simulink model "Auris_ES14"  (R2019a)
settings: Solver=FixedStepAuto  StartTime=0.0  StopTime=10000  FixedStep=.1  RelTol=1e-5
PostLoadFcn:
  | if builtin('license','test','virtual_reality_toolbox')
  |     set_param([gcs '/Simulink 3D Animation'], 'enableVis', 'on')
  | else
  |     set_param([gcs '/Simulink 3D Animation'], 'enableVis', 'off')
  | end
InitFcn:
  | if strcmp(get_param([gcs '/Simulink 3D Animation'], 'enableVis'), 'on')
  |     if ~builtin('license','checkout','virtual_reality_toolbox')
  |         error(message('aeroblks_cubesat:cubesat:licenseFailAnimTemplate'));
  |     end
  | end
model workspace (MATLAB code in the model file + MAT data in the model file):
  aeroCoeff : struct (value not decoded)
  environment : struct (value not decoded)
  initCond : struct (value not decoded)
  inputs0 : struct (value not decoded)
  states0 : struct (value not decoded)
  vehicle : struct (value not decoded)
  other statements: initialize6DOFSkyHogg;
values from neighbouring files (symbols this model uses):
  combine_x_std = sqrt(sum([combine_x_std, pos_unc].^2))    [Pointing_Budget.m]
  combine_y_std = sqrt(sum([combine_y_std, pos_unc].^2))    [Pointing_Budget.m]
  combine_z_std = sqrt(sum([combine_z_std, pos_unc].^2))    [Pointing_Budget.m]
  epoch = juliandate(tle.epoch.year, 1, 1) + tle.epoch.day * 86400    [ADC_Sim_init.m]
  inertia = inertia * conversion    [ADC_Sim_init.m]
  initial_ang_rate = [0, 0, 0]    [ADC_Sim_init.m]
  initial_euler = [0, 0, 180]    [ADC_Sim_init.m]
  s = line1(3:7)    [read_tloes.m]
  semi_major = (((86400 / tle.mean_motion) / (2 * pi))^2 * 398.6e12)^(1 / 3)    [ADC_Sim_init.m]
  starting_time = juliandate(date)    [ADC_Sim_init.m]
  tle = read_tloes('ISS_TLE.txt')    [ADC_Sim_init.m]
  true_anomaly = tle.mean_anomaly + (2 * exp(1) - 1 / 4 * exp(3)) * sind(tle.mean_anomaly) + 5 / 4 * exp(2) * sind(2 * tle.mean_anomaly) + 13/12 * exp(3) * sind(3 * tle.mean_anomaly)    [ADC_Sim_init.m]
undefined symbols (not defined in the file or in its folder): constraintAxes, Earth, euler0, IAU, km, pointing, pqr0, WGS84
libraries: aerolibutil x19, vrlib x8, aerolibconvert2 x6, sharedtransform x5, aerolibtransform2 x5, aerolibcelestial x3, asbCubeSatBlockLib x2, simulink x2, simulink_extras x2, aerolib6dof2 x1, sharedutil x1, aerolibobsolete x1
(part 2 of 2)

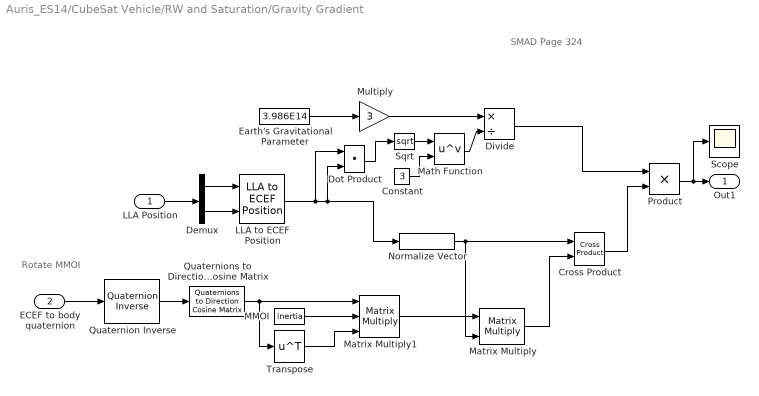
== system Auris_ES14/CubeSat Vehicle/RW and Saturation/Gravity Gradient ==
  note: SMAD Page 324
  note: Rotate MMOI
  LLA Position : Inport
  ECEF to body quaternion : Inport  Port=2
  Constant : Constant  Value=3
  Cross Product : vrlib/Utilities/Cross Product
      settings: SourceProductName=Simulink
  Demux : Demux  Outputs=2
  Divide : Product  Inputs=*/
  Dot Product : DotProduct  InputSameDT=on  OutDataTypeStr=Inherit: Inherit via internal rule
  Earth's Gravitational Parameter : Constant  Value=3.986E14
  LLA to ECEF Position : aerolibtransform2/LLA to ECEF Position  units=Metric (MKS)  ptype=Earth (WGS84)  F=1/298.257223563  R=6378137
      settings: SourceProductName=Aerospace Blockset  SourceProductBaseCode=AE
  MMOI : Constant  Value=inertia
  Math Function : Math  Operator=pow  SaturateOnIntegerOverflow=on
  Matrix Multiply : Product  Multiplication=Matrix(*)
  Matrix Multiply1 : Product  Inputs=3  Multiplication=Matrix(*)
  Multiply : Gain  Gain=3
  Normalize Vector : vrlib/Utilities/Normalize Vector  maxzero=0
      settings: SourceProductName=Simulink
  Product : Product
  Quaternion Inverse : aerolibutil/Quaternion Inverse
      settings: SourceProductName=Aerospace Blockset
  Quaternions to Direction Cosine Matrix : sharedtransform/Quaternions to  Direction Cosine Matrix  aMode=aMode
      settings: SourceProductName=Aerospace Blockset  SourceProductBaseCode=AE
  Scope : Scope
  Sqrt : Sqrt  SaturateOnIntegerOverflow=on
  Transpose : Math  Operator=transpose  SaturateOnIntegerOverflow=on
  Out1 : Outport
  wires:
  Demux/1 -> LLA to ECEF Position/1
  Demux/2 -> LLA to ECEF Position/2
  LLA Position/1 -> Demux/1
  Earth's Gravitational Parameter/1 -> Multiply/1
  LLA to ECEF Position/1 -> Normalize Vector/1, Dot Product/2, Dot Product/1
  Math Function/1 -> Divide/2
  Multiply/1 -> Divide/1
  Normalize Vector/1 -> Matrix Multiply/2, Cross Product/1
  Product/1 -> Scope/1, Out1/1
  Divide/1 -> Product/1
  Cross Product/1 -> Product/2
  Matrix Multiply/1 -> Cross Product/2
  ECEF to body quaternion/1 -> Quaternion Inverse/1
  Quaternion Inverse/1 -> Quaternions to Direction Cosine Matrix/1
  MMOI/1 -> Matrix Multiply1/2
  Quaternions to Direction Cosine Matrix/1 -> Transpose/1, Matrix Multiply1/1
  Transpose/1 -> Matrix Multiply1/3
  Matrix Multiply1/1 -> Matrix Multiply/1
  Dot Product/1 -> Sqrt/1
  Sqrt/1 -> Math Function/1
  Constant/1 -> Math Function/2

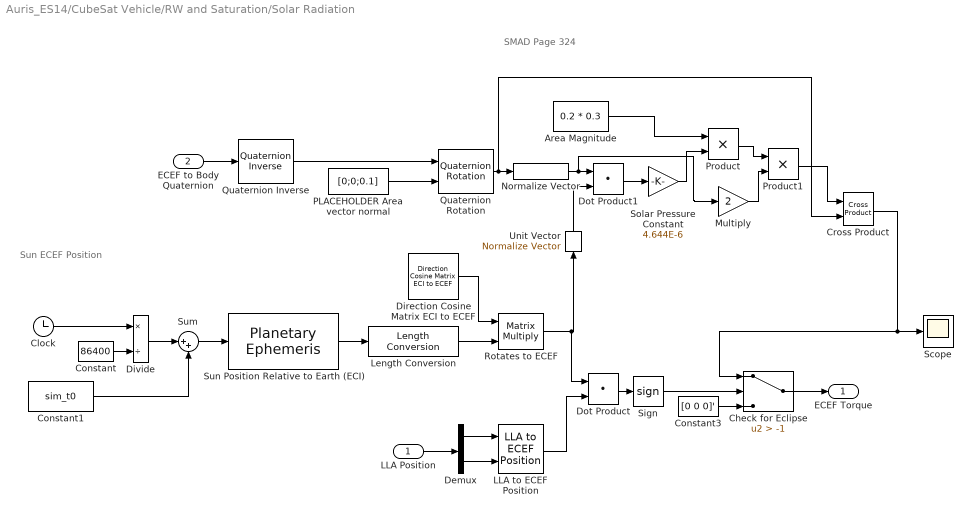
== system Auris_ES14/CubeSat Vehicle/RW and Saturation/Solar Radiation ==
  note: Sun ECEF Position
  note: SMAD Page 324
  LLA Position : Inport
  ECEF to Body Quaternion : Inport  Port=2
  "Area Magnitude " : Constant  Value=0.2 * 0.3
  Check for Eclipse : Switch  Criteria=u2 > Threshold  Threshold=-1
  Clock : Clock
  Constant : Constant  Value=86400
  Constant1 : Constant  Value=sim_t0
  Constant3 : Constant  Value=[0 0 0]'  OutDataTypeStr=Inherit: Inherit via back propagation
  Cross Product : vrlib/Utilities/Cross Product
      settings: SourceProductName=Simulink
  Demux : Demux  Outputs=2
  Direction Cosine Matrix ECI to ECEF : aerolibtransform2/Direction Cosine Matrix ECI to ECEF  red=IAU-2000/2006  year=2019  month=January  day=4  hour=0  min=0  sec=0  deltaT=None  errorflag=Error  extraparamflag=off
      settings: AttributesFormatString=%<red>  SourceProductName=Aerospace Blockset  SourceProductBaseCode=AE
  Divide : Product  Inputs=*/
  Dot Product : DotProduct  InputSameDT=on  OutDataTypeStr=Inherit: Inherit via internal rule
  Dot Product1 : DotProduct  InputSameDT=on  OutDataTypeStr=Inherit: Inherit via internal rule
  LLA to ECEF Position : aerolibtransform2/LLA to ECEF Position  units=Metric (MKS)  ptype=Earth (WGS84)  F=1/298.257223563  R=6378137
      settings: SourceProductName=Aerospace Blockset  SourceProductBaseCode=AE
  Length Conversion : aerolibconvert2/Length Conversion  IU=km  OU=m
  Multiply : Gain  Gain=2
  Normalize Vector : vrlib/Utilities/Normalize Vector  maxzero=0
      settings: SourceProductName=Simulink
  PLACEHOLDER Area vector normal : Constant  Value=[0;0;0.1]
  Product : Product
  Product1 : Product
  Quaternion Inverse : aerolibutil/Quaternion Inverse
      settings: SourceProductName=Aerospace Blockset
  Quaternion Rotation : aerolibutil/Quaternion Rotation
  Rotates to ECEF : Product  Multiplication=Matrix(*)
  Scope : Scope
  Sign : Signum
  Solar Pressure Constant : Gain  Gain=4.644E-6
  Sum : Sum  Inputs=|++
  Sun Position Relative to Earth (ECI) : aerolibcelestial/Planetary Ephemeris  kmflag=km,km/s  epochflag=Julian date  de=DE421  nCenter=Earth  nTarget=Sun  errorflag=Error  velflag=off
      settings: SourceProductName=Aerospace Blockset  SourceProductBaseCode=AE
  Unit Vector : vrlib/Utilities/Normalize Vector  maxzero=0
      settings: SourceProductName=Simulink
  ECEF Torque : Outport
  wires:
  Constant1/1 -> Sum/2
  Clock/1 -> Divide/1
  Constant/1 -> Divide/2
  Divide/1 -> Sum/1
  Sum/1 -> Sun Position Relative to Earth (ECI)/1
  Sun Position Relative to Earth (ECI)/1 -> Length Conversion/1
  Direction Cosine Matrix ECI to ECEF/1 -> Rotates to ECEF/1
  Length Conversion/1 -> Rotates to ECEF/2
  LLA Position/1 -> Demux/1
  Demux/1 -> LLA to ECEF Position/1
  Demux/2 -> LLA to ECEF Position/2
  Rotates to ECEF/1 -> Unit Vector/1, Dot Product/1
  LLA to ECEF Position/1 -> Dot Product/2
  Check for Eclipse/1 -> ECEF Torque/1
  Constant3/1 -> Check for Eclipse/3
  Normalize Vector/1 -> Multiply/1, Dot Product1/1
  Dot Product1/1 -> Solar Pressure Constant/1
  Quaternion Rotation/1 -> Cross Product/2, Normalize Vector/1
  PLACEHOLDER Area vector normal/1 -> Quaternion Rotation/2
  ECEF to Body Quaternion/1 -> Quaternion Inverse/1
  Quaternion Inverse/1 -> Quaternion Rotation/1
  Unit Vector/1 -> Dot Product1/2
  Solar Pressure Constant/1 -> Product/2
  "Area Magnitude "/1 -> Product/1
  Product/1 -> Product1/1
  Multiply/1 -> Product1/2
  Product1/1 -> Cross Product/1
  Dot Product/1 -> Sign/1
  Sign/1 -> Check for Eclipse/2
  Cross Product/1 -> Check for Eclipse/1, Scope/1

== system Auris_ES14/Simulink 3D Animation/Antenna Position to VRML/ECEF to VRML ==
  M : Inport  PortDimensions=3
  Demux : Demux  Outputs=3
  Gain3 : Gain  Gain=-1
  Mux : Mux  Inputs=3
  VR : Outport  PortDimensions=3
  wires:
  M/1 -> Demux/1
  Demux/1 -> Gain3/1
  Demux/2 -> Mux/3
  Demux/3 -> Mux/2
  Mux/1 -> VR/1
  Gain3/1 -> Mux/1

== system Auris_ES14/Simulink 3D Animation/Compute Earth Rotation Rate/Quaternion to VRML ==
  q : Inport
  Demux : Demux
  Gain : Gain  Gain=2
  Gain3 : Gain  Gain=[-1 1 1 1]
  Mux : Mux
  Selector : Selector  InputPortWidth=4  IndexOptions=Index vector (dialog)  Indices=[2 4 3 1]  OutputSizes=1
  Trigonometric Function : Trigonometry  Operator=acos
  AxisAngle : Outport
  wires:
  Demux/1 -> Trigonometric Function/1
  Trigonometric Function/1 -> Gain/1
  Mux/1 -> Selector/1
  q/1 -> Demux/1
  Gain3/1 -> AxisAngle/1
  Selector/1 -> Gain3/1
  Gain/1 -> Mux/1
  Demux/2 -> Mux/2
  Demux/3 -> Mux/3
  Demux/4 -> Mux/4

== system Auris_ES14/Simulink 3D Animation/Compute Umbra Translation/unitVec ==
  I : Inport
  Divide : Product  Inputs=*/
  Dot Product : DotProduct  InputSameDT=on  OutDataTypeStr=Inherit: Inherit via internal rule
  Sqrt : Sqrt  SaturateOnIntegerOverflow=on
  O : Outport
  wires:
  Dot Product/1 -> Sqrt/1
  I/1 -> Divide/1, Dot Product/1, Dot Product/2
  Divide/1 -> O/1
  Sqrt/1 -> Divide/2

== system Auris_ES14/Simulink 3D Animation/Sat Position to VRML/ECEF to VRML ==
  M : Inport  PortDimensions=3
  Demux : Demux  Outputs=3
  Gain3 : Gain  Gain=-1
  Mux : Mux  Inputs=3
  VR : Outport  PortDimensions=3
  wires:
  M/1 -> Demux/1
  Demux/1 -> Gain3/1
  Demux/2 -> Mux/3
  Demux/3 -> Mux/2
  Mux/1 -> VR/1
  Gain3/1 -> Mux/1

== system Auris_ES14/Simulink 3D Animation/Sun Position to VRML/ECEF to VRML ==
  M : Inport  PortDimensions=3
  Demux : Demux  Outputs=3
  Gain3 : Gain  Gain=-1
  Mux : Mux  Inputs=3
  VR : Outport  PortDimensions=3
  wires:
  M/1 -> Demux/1
  Demux/1 -> Gain3/1
  Demux/2 -> Mux/3
  Demux/3 -> Mux/2
  Mux/1 -> VR/1
  Gain3/1 -> Mux/1

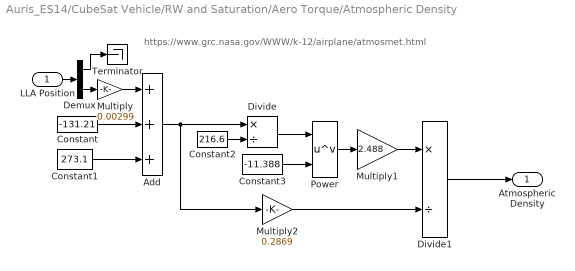
== system Auris_ES14/CubeSat Vehicle/RW and Saturation/Aero Torque/Atmospheric Density ==
  note: https://www.grc.nasa.gov/WWW/k-12/airplane/atmosmet.html
  LLA Position : Inport
  Add : Sum  Inputs=+++
  Constant : Constant  Value=-131.21
  Constant1 : Constant  Value=273.1
  Constant2 : Constant  Value=216.6
  Constant3 : Constant  Value=-11.388
  Demux : Demux  Outputs=2
  Divide : Product  Inputs=*/
  Divide1 : Product  Inputs=*/
  Multiply : Gain  Gain=0.00299
  Multiply1 : Gain  Gain=2.488
  Multiply2 : Gain  Gain=0.2869
  Power : Math  Operator=pow  SaturateOnIntegerOverflow=on
  Terminator : Terminator
  Atmospheric Density : Outport
  wires:
  LLA Position/1 -> Demux/1
  Demux/1 -> Terminator/1
  Constant/1 -> Add/2
  Multiply/1 -> Add/1
  Demux/2 -> Multiply/1
  Constant1/1 -> Add/3
  Add/1 -> Multiply2/1, Divide/1
  Constant2/1 -> Divide/2
  Divide/1 -> Power/1
  Constant3/1 -> Power/2
  Power/1 -> Multiply1/1
  Multiply1/1 -> Divide1/1
  Multiply2/1 -> Divide1/2
  Divide1/1 -> Atmospheric Density/1
